simulink model "Design"  (R2022b)
settings: Solver=VariableStepAuto  StartTime=0.0  StopTime=10.0  RelTol=1e-3
libraries: cstblocks x8
settings Model: Creator=antoninrenoir  LastModifiedBy=antoninrenoir

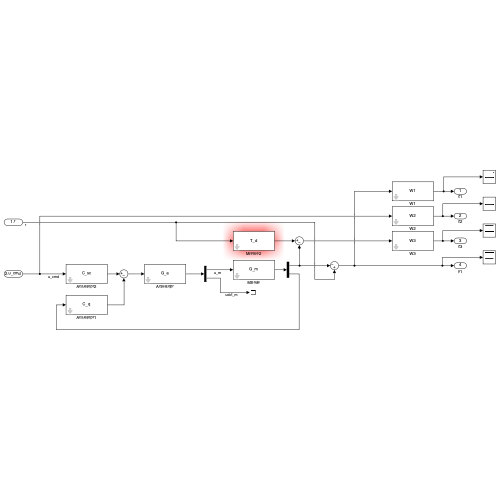
[thumbnail: Simulink's stored preview of the top-level diagram]
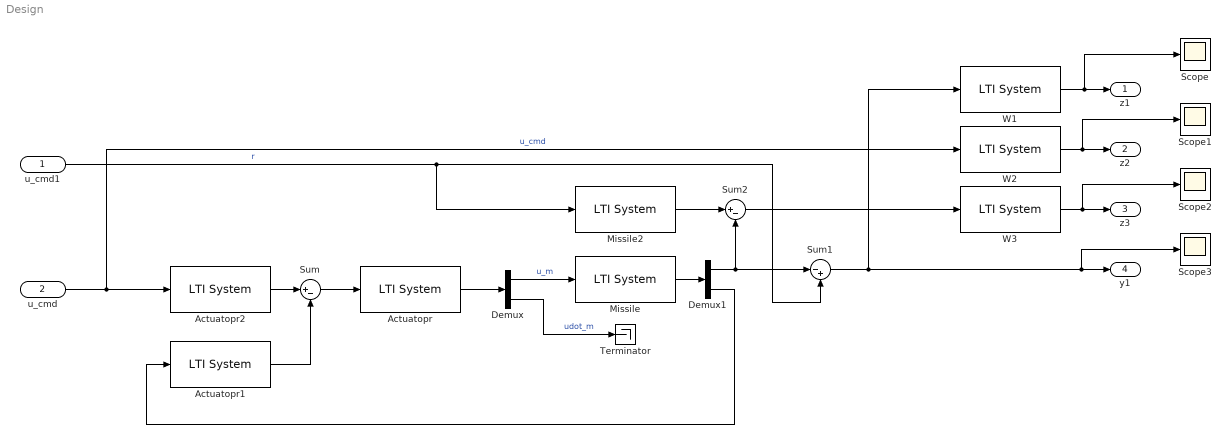
== system Design ==
  u_cmd1 : Inport
  u_cmd : Inport  Port=2
  Actuatopr : cstblocks/LTI System  sys=G_a  IC=[]
  Actuatopr1 : cstblocks/LTI System  sys=C_q  IC=[]
  Actuatopr2 : cstblocks/LTI System  sys=C_sc  IC=[]
  Demux : Demux  Outputs=2
  Demux1 : Demux  Outputs=2
  Missile : cstblocks/LTI System  sys=G_m  IC=[]
  Missile2 : cstblocks/LTI System  sys=T_d  IC=[]
  Scope{,1..3} (4 alike) : Scope
  Sum : Sum  Inputs=|+-
  Sum1 : Sum  Inputs=|-+
  Sum2 : Sum  Inputs=|+-
  Terminator : Terminator
  W1 : cstblocks/LTI System  sys=W1  IC=[]
  W2 : cstblocks/LTI System  sys=W2  IC=[]
  W3 : cstblocks/LTI System  sys=W3  IC=[]
  z1 : Outport
  z2 : Outport  Port=2
  z3 : Outport  Port=3
  y1 : Outport  Port=4
  wires:
  Missile/1 -> Demux1/1
  Actuatopr/1 -> Demux/1
  u_cmd/1 -> W2/1, Actuatopr2/1  "u_cmd"
  Actuatopr2/1 -> Sum/1
  Demux/1 -> Missile/1  "u_m"
  Demux/2 -> Terminator/1  "udot_m"
  Actuatopr1/1 -> Sum/2
  Demux1/2 -> Actuatopr1/1
  Sum/1 -> Actuatopr/1
  Demux1/1 -> Sum2/2, Sum1/1
  Sum1/1 -> W1/1, Scope3/1, y1/1
  u_cmd1/1 -> Missile2/1, Sum1/2  "r"
  Missile2/1 -> Sum2/1
  W2/1 -> Scope1/1, z2/1
  W1/1 -> Scope/1, z1/1
  Sum2/1 -> W3/1
  W3/1 -> Scope2/1, z3/1
